simulink model "RobotDoSrodka10cmSim"  (R2018a)
settings: Solver=ode45  StartTime=0.0  StopTime=tsym  RelTol=1e-6
values from neighbouring files (symbols this model uses):
  k1 = 1    [RobotDoSrodka10cm.m]
  k2 = 10    [RobotDoSrodka10cm.m]
  l = 0.095    [RobotDoSrodka10cm.m]
  R = 0.034    [RobotDoSrodka10cm.m]
undefined symbols (not defined in the file or in its folder): wd
settings Model: Creator=Papa Smerf  LastModifiedBy=Papa Smerf
settings DataIOCC: LimitDataPoints=on  SaveFormat=Array
settings OptimizationCC: BlockReduction=off  BooleanDataType=off  LifeSpan=inf
settings DebuggingCC: SaveWithParameterizedLinksMsg=none  UnderspecifiedInitializationDetection=Classic  MergeDetectMultiDrivingBlocksExec=none  SignalResolutionControl=TryResolveAllWithWarning  SFUnexpectedBacktrackingDiag=warning  SFNoUnconditionalDefaultTransitionDiag=warning  SFExecutionAtInitializationDiag=none
settings HardwareCC: ProdBitPerPointer=32  ProdBitPerSizeT=32  ProdBitPerPtrDiffT=32  ProdLargestAtomicFloat=None  ProdIntDivRoundTo=Undefined  ProdEndianess=Unspecified  ProdWordSize=32  ProdHWDeviceType=32-bit Generic  TargetUnknown=on
settings ModelReferenceCC: PropagateSignalLabelsOutOfModel=off
settings CodeAppCC: StateflowObjectComments=on
settings GRTTargetCC: TargetLangStandard=C89/C90 (ANSI)  GeneratePreprocessorConditionals=Disable all
settings ConfigComp: CovMetricSettings=dw  CovHtmlReporting=on  CovSaveCumulativeToWorkspaceVar=on  CovSaveSingleToWorkspaceVar=on  CovExternalEMLEnable=off  CovSFcnEnable=off

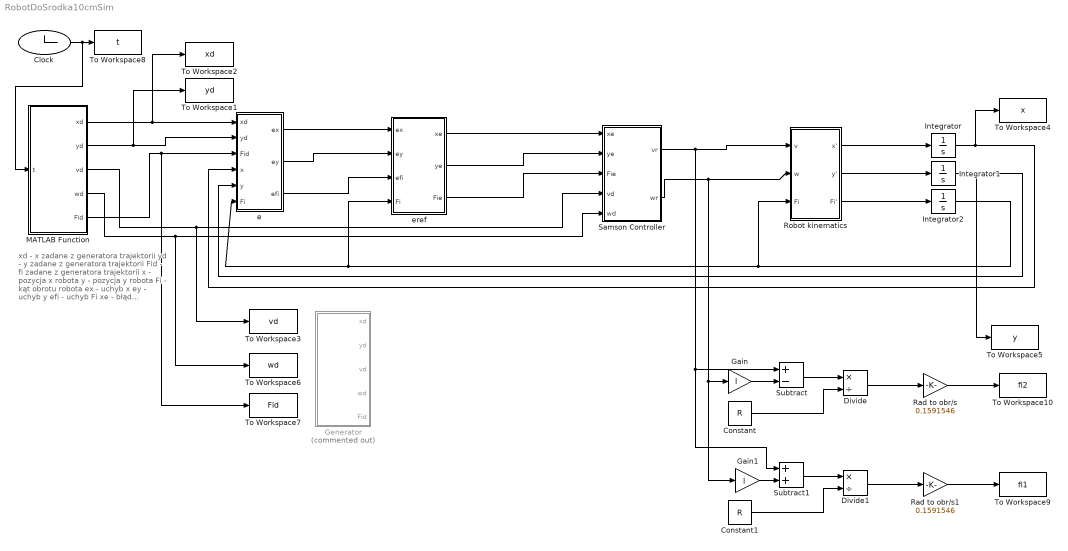
== system RobotDoSrodka10cmSim ==
  note: xd - x zadane z generatora trajektorii
      | yd - y zadane z generatora trajektorii
      | Fid - fi zadane z generatora trajektorii
      | x - pozycja x robota
      | y - pozycja y robota
      | Fi - kąt obrotu robota
      | ex - uchyb x
      | ey - uchyb y
      | efi - uchyb Fi
      | xe - błąd referencyjny x
      | ye - błąd referencyjny y
      | Fie - błąd referencyjny Fi
      | vd - prędkość liniowa zadana
      | wd - prędkość kątowa zadana
      | vr - prędkość liniowa referencyjna
      | wr - prędkość kątowa referencyjna
      | v - prędkość liniowa zadana robota?
      | w - prędkość kątowa zadana robota?
      | x' - prędkość w osi x robota
      | y' - prędkość w osi y robota
      | Fi' - prędkość kątowa robota
  Clock : Clock
  Constant : Constant  Value=R
  Constant1 : Constant  Value=R
  Divide : Product  Inputs=*/
  Divide1 : Product  Inputs=*/
  Gain : Gain  Gain=l
  Gain1 : Gain  Gain=l
  Generator : Subsystem  Commented=on
  Integrator : Integrator
  Integrator1 : Integrator
  Integrator2 : Integrator
  MATLAB Function : MATLAB Function  TreatAsAtomicUnit=on
  Rad to obr/s : Gain  Gain=0.1591546
  Rad to obr/s1 : Gain  Gain=0.1591546
  Robot kinematics : Subsystem
  Samson Controller : Subsystem
  Subtract : Sum  Inputs=+-
  Subtract1 : Sum
  To Workspace1 : ToWorkspace  VariableName=yd  SampleTime=-1
  To Workspace10 : ToWorkspace  VariableName=fi2  SampleTime=0.01
  To Workspace2 : ToWorkspace  VariableName=xd  SampleTime=-1
  To Workspace3 : ToWorkspace  VariableName=vd  SampleTime=-1
  To Workspace4 : ToWorkspace  VariableName=x  SampleTime=-1
  To Workspace5 : ToWorkspace  VariableName=y  SampleTime=-1
  To Workspace6 : ToWorkspace  VariableName=wd  SampleTime=-1
  To Workspace7 : ToWorkspace  VariableName=Fid  SampleTime=-1
  To Workspace8 : ToWorkspace  VariableName=t  SampleTime=0.01
  To Workspace9 : ToWorkspace  VariableName=fi1  SampleTime=0.01
  e : Subsystem
  eref : Subsystem
  wires:
  e/1(ex) -> eref/1(ex)
  e/2(ey) -> eref/2(ey)
  e/3(efi) -> eref/3(efi)
  eref/1(xe) -> Samson Controller/1(xe)
  eref/2(ye) -> Samson Controller/2(ye)
  eref/3(Fie) -> Samson Controller/3(Fie)
  Robot kinematics/1(x') -> Integrator/1
  Robot kinematics/2(y') -> Integrator1/1
  Robot kinematics/3(Fi') -> Integrator2/1
  Integrator2/1 -> Robot kinematics/3(Fi), e/6(Fi), eref/4(Fi)
  Integrator1/1 -> To Workspace5/1, e/5(y)
  Integrator/1 -> To Workspace4/1, e/4(x)
  MATLAB Function/1(xd) -> To Workspace2/1, e/1(xd)
  MATLAB Function/2(yd) -> To Workspace1/1, e/2(yd)
  MATLAB Function/5(Fid) -> To Workspace7/1, e/3(Fid)
  MATLAB Function/3(vd) -> To Workspace3/1, Samson Controller/4(vd)
  MATLAB Function/4(wd) -> To Workspace6/1, Samson Controller/5(wd)
  Clock/1 -> MATLAB Function/1(t), To Workspace8/1
  Rad to obr/s1/1 -> To Workspace9/1
  Divide1/1 -> Rad to obr/s1/1
  Divide/1 -> Rad to obr/s/1
  Gain1/1 -> Subtract1/2
  Gain/1 -> Subtract/2
  Subtract1/1 -> Divide1/1
  Constant1/1 -> Divide1/2
  Samson Controller/1(vr) -> Subtract1/1, Subtract/1, Robot kinematics/1(v)
  Constant/1 -> Divide/2
  Samson Controller/2(wr) -> Gain1/1, Gain/1, Robot kinematics/2(w)
  Subtract/1 -> Divide/1
  Rad to obr/s/1 -> To Workspace10/1

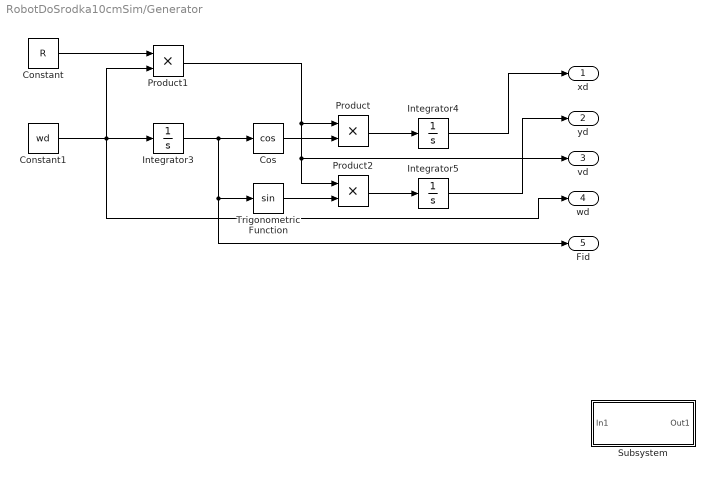
== system RobotDoSrodka10cmSim/Generator ==
  Constant : Constant  Value=R
  Constant1 : Constant  Value=wd
  Cos : Trigonometry  Operator=cos
  Integrator3 : Integrator
  Integrator4 : Integrator
  Integrator5 : Integrator  InitialCondition=-R
  Product : Product
  Product1 : Product
  Product2 : Product
  Subsystem : Subsystem
  Trigonometric Function : Trigonometry
  xd : Outport
  yd : Outport  Port=2
  vd : Outport  Port=3
  wd : Outport  Port=4
  Fid : Outport  Port=5
  wires:
  Integrator5/1 -> yd/1
  Product1/1 -> vd/1, Product2/1, Product/1
  Constant/1 -> Product1/1
  Integrator3/1 -> Fid/1, Trigonometric Function/1, Cos/1
  Trigonometric Function/1 -> Product2/2
  Product/1 -> Integrator4/1
  Constant1/1 -> wd/1, Product1/2, Integrator3/1
  Cos/1 -> Product/2
  Integrator4/1 -> xd/1
  Product2/1 -> Integrator5/1

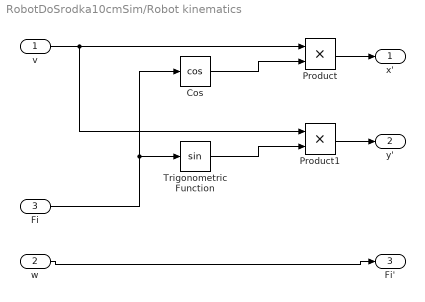
== system RobotDoSrodka10cmSim/Robot kinematics ==
  v : Inport
  w : Inport  Port=2
  Fi : Inport  Port=3
  Cos : Trigonometry  Operator=cos
  Product : Product
  Product1 : Product
  Trigonometric Function : Trigonometry
  x' : Outport
  y' : Outport  Port=2
  Fi' : Outport  Port=3
  wires:
  w/1 -> Fi'/1
  Fi/1 -> Cos/1, Trigonometric Function/1
  Product1/1 -> y'/1
  v/1 -> Product1/1, Product/1
  Cos/1 -> Product/2
  Product/1 -> x'/1
  Trigonometric Function/1 -> Product1/2

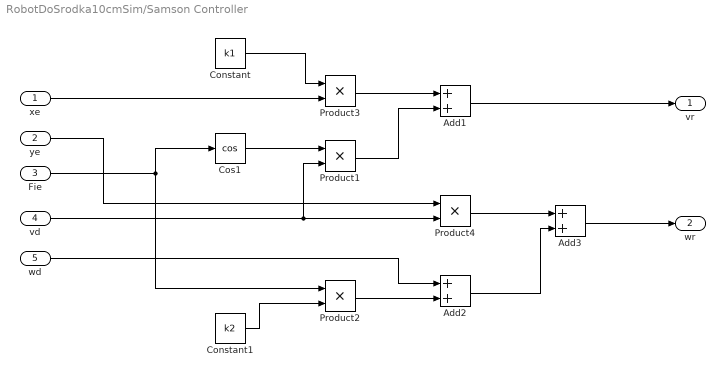
== system RobotDoSrodka10cmSim/Samson Controller ==
  xe : Inport
  ye : Inport  Port=2
  Fie : Inport  Port=3
  vd : Inport  Port=4
  wd : Inport  Port=5
  Add1 : Sum
  Add2 : Sum
  Add3 : Sum
  Constant : Constant  Value=k1
  Constant1 : Constant  Value=k2
  Cos1 : Trigonometry  Operator=cos
  Product{1..4} (4 alike) : Product
  vr : Outport
  wr : Outport  Port=2
  wires:
  ye/1 -> Product4/1
  Fie/1 -> Product2/1, Cos1/1
  vd/1 -> Product4/2, Product1/2
  Add2/1 -> Add3/2
  Cos1/1 -> Product1/1
  xe/1 -> Product3/2
  Product3/1 -> Add1/1
  Product2/1 -> Add2/2
  Product1/1 -> Add1/2
  Add3/1 -> wr/1
  Add1/1 -> vr/1
  Constant/1 -> Product3/1
  Constant1/1 -> Product2/2
  wd/1 -> Add2/1
  Product4/1 -> Add3/1

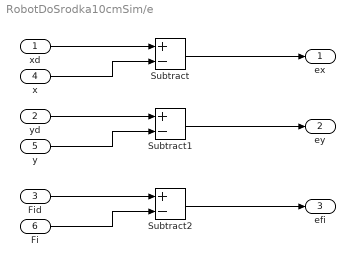
== system RobotDoSrodka10cmSim/e ==
  xd : Inport
  yd : Inport  Port=2
  Fid : Inport  Port=3
  x : Inport  Port=4
  y : Inport  Port=5
  Fi : Inport  Port=6
  Subtract : Sum  Inputs=+-
  Subtract1 : Sum  Inputs=+-
  Subtract2 : Sum  Inputs=+-
  ex : Outport
  ey : Outport  Port=2
  efi : Outport  Port=3
  wires:
  Subtract/1 -> ex/1
  xd/1 -> Subtract/1
  Fi/1 -> Subtract2/2
  x/1 -> Subtract/2
  Subtract2/1 -> efi/1
  Fid/1 -> Subtract2/1
  Subtract1/1 -> ey/1
  yd/1 -> Subtract1/1
  y/1 -> Subtract1/2

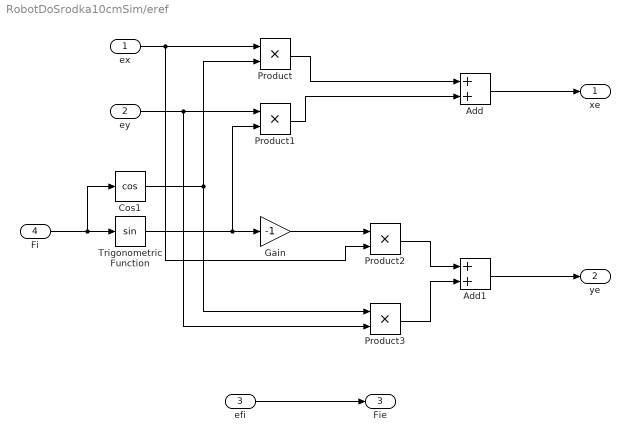
== system RobotDoSrodka10cmSim/eref ==
  ex : Inport
  ey : Inport  Port=2
  efi : Inport  Port=3
  Fi : Inport  Port=4
  Add : Sum
  Add1 : Sum
  Cos1 : Trigonometry  Operator=cos
  Gain : Gain  Gain=-1
  Product{,1..3} (4 alike) : Product
  Trigonometric Function : Trigonometry
  xe : Outport
  ye : Outport  Port=2
  Fie : Outport  Port=3
  wires:
  Cos1/1 -> Product3/1, Product/2
  Product1/1 -> Add/2
  ey/1 -> Product3/2, Product1/1
  Add/1 -> xe/1
  Trigonometric Function/1 -> Product1/2, Gain/1
  Fi/1 -> Cos1/1, Trigonometric Function/1
  Product3/1 -> Add1/2
  Product/1 -> Add/1
  Add1/1 -> ye/1
  ex/1 -> Product2/2, Product/1
  Gain/1 -> Product2/1
  efi/1 -> Fie/1
  Product2/1 -> Add1/1

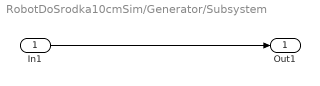
== system RobotDoSrodka10cmSim/Generator/Subsystem ==
  In1 : Inport
  Out1 : Outport
  wires:
  In1/1 -> Out1/1

== matlab function RobotDoSrodka10cmSim/MATLAB Function ==
  data: t input; xd output; yd output; vd output; wd output; Fid output
function [xd, yd, vd, wd, Fid] = fcn(t)

xd=0;
yd=0;
Fid=0;
vd=0.1;
wd=0;

if t<=10
    xd=vd*t;
    yd=0;
    Fid=0;
elseif ((t>10) && (t<=20))
    xd=1;
    yd=(vd*t-1);
    Fid=pi/2;
elseif ((t>20) && (t<=30))
    xd=1-(vd*t-2);
    yd=1;
    Fid=pi;
elseif ((t>30) && (t<=38))
    xd=0;
    yd=1-(vd*t-3);
    Fid=3/2*pi;
elseif ((t>38) && (t<=46))
    xd=vd*t-3.8;
    yd=0.2;
    Fid=0;   
elseif ((t>46) && (t<=52))
    xd= 0.8;
    yd= 0.2 +(vd*t-4.6);
    Fid=pi/2;
elseif ((t>52) && (t<=58))
    xd=0.8-(vd*t-5.2);
    yd=0.8;
    Fid=pi;
elseif ((t>58) && (t<=62))
    xd=0.2;
    yd=0.8-(vd*t-5.8);
    Fid=3/2*pi;
elseif ((t>62) && (t<=66))
    xd=0.2 + vd*t-6.2;
    yd=0.4;
    Fid=0;  
elseif ((t>66) && (t<=68))
    xd= 0.6;
    yd= 0.4 +(vd*t-6.6);
    Fid=pi/2;
elseif ((t>68) && (t<=70))
    xd=0.6-(vd*t-6.8);
    yd=0.6;
    Fid=pi;
elseif (t>70)
    xd=0.4;
    yd=0.6;
    Fid=pi;
end
